simulink model "sl_lanechange"  (R2022a)
settings: Solver=ode45  StartTime=0.0  StopTime=10.0  RelTol=1e-3  EnableMultiTasking=on
libraries: robotmobilelib x1, simulink x1
Description:
  | Simple lane changing maneuver.
  | The pulse generator drives the steered angle left, then right.
  | 
  | Robotics, Vision and Control - 3rd Edition; Section 4.1.1
settings Model: Creator=pic  LastModifiedBy=rpill
settings SolverCC: AlgebraicLoopSolver=TrustRegion  MaxZcPerStep=1
settings DataIOCC: LimitDataPoints=on  SaveFormat=Array  SignalLoggingSaveFormat=ModelDataLogs  DSMLogging=off  VisualizeSimOutput=off  TimeSaveName=t  OutputSaveName=y
settings OptimizationCC: ExpressionDepthLimit=2147483647  LifeSpan=inf
settings DebuggingCC: UnderspecifiedInitializationDetection=Classic  MergeDetectMultiDrivingBlocksExec=none  SolverPrmCheckMsg=warning  FcnCallInpInsideContextMsg=warning  UnconnectedInputMsg=warning  UnconnectedOutputMsg=warning  UnconnectedLineMsg=warning  AllowSymbolicDim=off  StateNameClashWarn=warning  SFUnexpectedBacktrackingDiag=warning  SFNoUnconditionalDefaultTransitionDiag=warning  SFMachineParentedDataDiag=warning  ArithmeticOperatorsInVariantConditions=warning
settings HardwareCC: ProdBitPerPointer=32  ProdBitPerSizeT=32  ProdBitPerPtrDiffT=32  ProdLargestAtomicFloat=None  ProdIntDivRoundTo=Undefined  ProdEndianess=Unspecified  ProdWordSize=32  ProdHWDeviceType=32-bit Generic
settings ModelReferenceCC: PropagateSignalLabelsOutOfModel=off
settings SFSimCC: SimUseLocalCustomCode=off  CustomCodeUndefinedFunction=UseInterfaceOnly
settings RTWCC: RTWUseLocalCustomCode=off  DLArmComputeVersion=19.05
settings CodeAppCC: StateflowObjectComments=on
settings GRTTargetCC: TargetLangStandard=C89/C90 (ANSI)  CombineOutputUpdateFcns=off  GRTInterface=on
settings ConfigComp: CovMetricSettings=dw  CovSaveCumulativeToWorkspaceVar=on  CovSaveSingleToWorkspaceVar=on  CovExternalEMLEnable=off

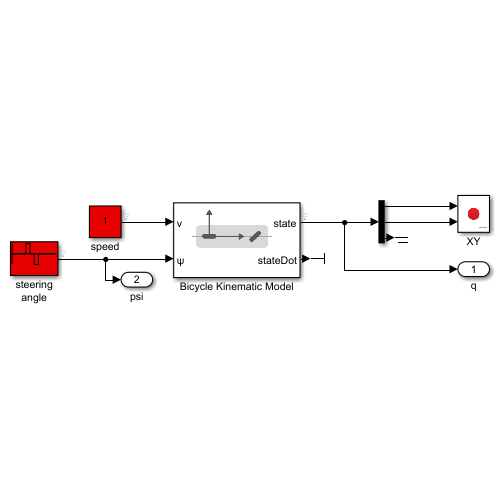
[thumbnail: Simulink's stored preview of the top-level diagram]
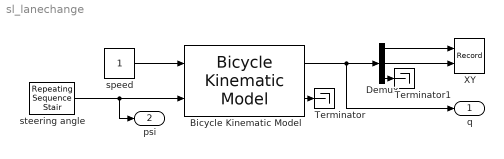
== system sl_lanechange ==
  Bicycle Kinematic Model : robotmobilelib/Bicycle Kinematic Model  VehicleInputs=Vehicle Speed & Steering Angle  WheelBase=1  VehicleSpeedRange=[0 1]  MaxSteeringAngle=2  InitialState=[0; 0; 0]  SimulateUsing=Interpreted execution
      settings: SourceProductBaseCode=RO
  Demux : Demux  Outputs=3
  Terminator : Terminator
  Terminator1 : Terminator
  XY : Record  FileSettingsInternal="{\"entries\":[{\"content\":{\"excelSettings\":{\"content\":{},\"type\":\"Streamout.ExcelSettings\"}},\"type\":\"Streamout.FileSettingStorage\",\"uuid\":\"0d339c50-37b1-436a-8aad-213453601016\"}],\"packageUris\":[\"http://schema.mathworks.com/mf0/streamout_blocks/R2020a\"],\"version\":\"1.0\"}"  Layout=[1 1]  SignalsInternal="{\"entries\":[{\"content\":{\"signals\":[{\"content\":{\"blockPath\":[\"sl_lanechange/XY\"],\"channel\":[],\"dimensions\":[1],\"domain\":\"sl_lanechange/XY\",\"lineColor\":\"#a2142f\",\"plots\":[1],\"port\":1,\"sid\":[],\"signalID\":9,\"signalName\":\"XY Graph:1\"},\"type\":\"RecordBlkView.Signal\",\"uuid\":\"8d1f29f8-04ba-495f-9965-6860bc0c8a6b\"},{\"content\":{\"blockPath\":[\"sl_lanechange/XY\"],\"channel\":[],\"dimensions\":[1],\"domain\":\"sl_lanechange/XY\",\"lineColor\":\"#139fff\",\"plots\":[1],\"port\":2,\"sid\":[],\"signalID\":12,\"signalName\":\"XY Graph:2\"},\"type\":\"RecordBlkView.Signal\",\"uuid\":\"1fd1b70e-1376-41b6-844b-bf0b26112049\"}]},\"type\":\"RecordBlkView.InputSignals\",\"uuid\":\"854d0c3b-bb39-4ebe-a254-602af473da18\"}],\"packageUris\":[\"http://schema.mathworks.com/mf0/streamout_blocks/R2020a\"],\"version\":\"1.0\"}"  VisualizationBindings="{\"xyplotplugin\":{\"info\":[{\"series\":[{\"bindingParametersList\":[{\"parameter\":\"X-Axis\",\"signalID\":9,\"signalName\":\"XY Graph:1\"},{\"parameter\":\"Y-Axis\",\"signalID\":12,\"signalName\":\"XY Graph:2\"}],\"seriesID\":43401}],\"subplotID\":1}]}}"  CompatibilityTag=XY  st=-1
  speed : Constant  VectorParams1D=off  SampleTime=0.02
  steering angle : simulink/Sources/Repeating Sequence Stair  OutValues=[0 0 0 0.5 0 -0.5 0 0 0 0]  tsamp=1  OutMin=[]  OutMax=[]  OutDataTypeStr=double  OutputDataTypeScalingMode=Specify via dialog  OutDataType=double  ConRadixGroup=Best Precision: Vector-wise  OutScaling=2^-12
  q : Outport
  psi : Outport  Port=2
  wires:
  steering angle/1 -> Bicycle Kinematic Model/2, psi/1
  speed/1 -> Bicycle Kinematic Model/1
  Demux/1 -> XY/1
  Demux/2 -> XY/2
  Bicycle Kinematic Model/1 -> q/1, Demux/1
  Bicycle Kinematic Model/2 -> Terminator/1
  Demux/3 -> Terminator1/1
